simulink model "FIR_Symmetric_Ex2"  (R2025a)
settings: Solver=VariableStepAuto  StartTime=0.0  StopTime=1  RelTol=1e-3
PostLoadFcn:
  | Fs = 100000;  % Sampling Frequency
  | Fpass = 4000;              % Passband Frequency
  | Fstop = 10000;             % Stopband Frequency
  | Dpass = 0.0046051376314;   % Passband Ripple
  | Dstop = 0.00025118864315;  % Stopband Attenuation
  | dens  = 16;                % Density Factor
  | % Calculate the order from the parameters using FIRPMORD.
  | [N, Fo, Ao, W] = firpmord([Fpass, Fstop]/(Fs/2), [1 0], [Dpass, Dstop]);
  | % Calculate the coefficients using the FIRPM function.
  | coeffs = firpm(N, Fo, Ao, W, {dens});
InitFcn:
  | Fs = 100000;  % Sampling Frequency
  | Fpass = 4000;              % Passband Frequency
  | Fstop = 10000;             % Stopband Frequency
  | Dpass = 0.0046051376314;   % Passband Ripple
  | Dstop = 0.00025118864315;  % Stopband Attenuation
  | dens  = 16;                % Density Factor
  | % Calculate the order from the parameters using FIRPMORD.
  | [N, Fo, Ao, W] = firpmord([Fpass, Fstop]/(Fs/2), [1 0], [Dpass, Dstop]);
  | % Calculate the coefficients using the FIRPM function.
  | coeffs = firpm(N, Fo, Ao, W, {dens});
undefined symbols (not defined in the file): firpmord, None, S, vsva2197, xcvc1902
libraries: aieDSP x1, dspsrcs4 x1, dspmlti4 x1, vmcUtilities x1
settings Model: Creator=robg  LastModifiedBy=robg
settings DebuggingCC: UnconnectedInputMsg=warning  UnconnectedOutputMsg=warning  UnconnectedLineMsg=warning
settings ModelReferenceCC: EnableRefExpFcnMdlSchedulingChecks=on
settings RTWCC: GPUComputeCapability=3.5  DLArmComputeVersion=19.05

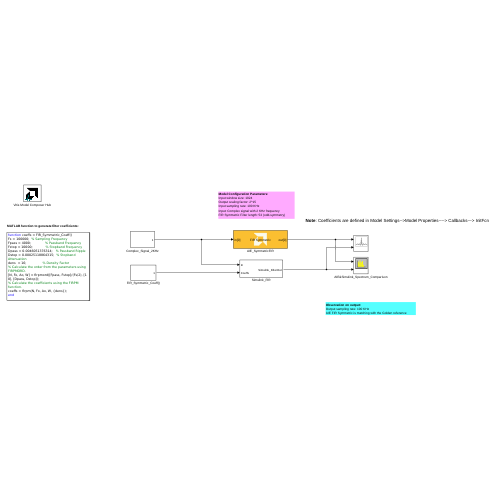
[thumbnail: Simulink's stored preview of the top-level diagram]
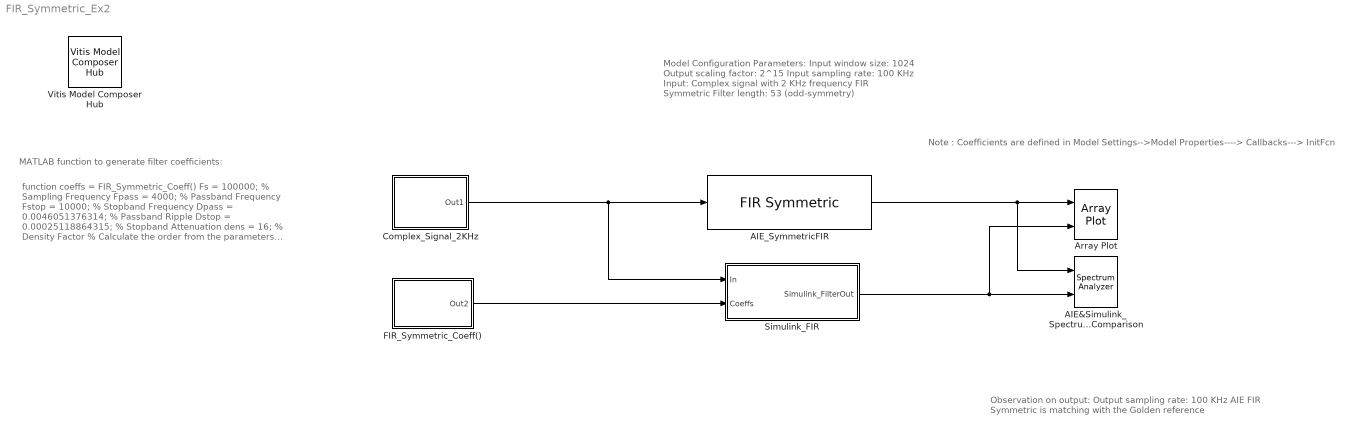
== system FIR_Symmetric_Ex2 ==
  note: Note : Coefficients are defined in Model Settings-->Model Properties----> Callbacks---> InitFcn
  note: Observation on output:
      | Output sampling rate: 100 KHz
      | AIE FIR Symmetric is matching with the Golden reference
  note: Model Configuration Parameters:
      | Input window size: 1024
      | Output scaling factor: 2^15
      | Input sampling rate: 100 KHz
      | Input: Complex signal with 2 KHz frequency
      | FIR Symmetric Filter length: 53 (odd-symmetry)
  note: MATLAB function to generate filter coefficients:
  note: function coeffs = FIR_Symmetric_Coeff()
      | Fs = 100000; % Sampling Frequency
      | Fpass = 4000; % Passband Frequency
      | Fstop = 10000; % Stopband Frequency
      | Dpass = 0.0046051376314; % Passband Ripple
      | Dstop = 0.00025118864315; % Stopband Attenuation
      | dens = 16; % Density Factor
      | % Calculate the order from the parameters using FIRPMORD.
      | [N, Fo, Ao, W] = firpmord([Fpass, Fstop]/(Fs/2), [1 0], [Dpass, Dstop]);
      | % Calculate the coefficients using the FIRPM function.
      | coeffs = firpm(N, Fo, Ao, W, {dens});
      | end
  AIE&Simulink_Spectrum_Comparison : SpectrumAnalyzer  NumInputPorts=2  WindowPosition=[439.000000,381.000000,800.000000,500.000000,]  Visible=on  ScopeFrameLocation=window  Span=99999.99999999999  StartFrequency=-49999.99999999999  StopFrequency=49999.99999999999  AveragingMethod=Exponential  YLimits=[-4.47944505,122.1232277]  ShowLegend=on  ChannelNames="[\"\"]"  AllowFFTLengthLessThanSamplesPerUpdate=on  DefaultConfigurationName=spbscopes.SpectrumAnalyzerBlockCfg
  AIE_SymmetricFIR : aieDSP/FIR Symmetric  data_type=cint16  coef_type=int16  use_coeff_reload=off  dual_ip=off  num_outputs=off  coeff=int16(coeffs(1:27)*2^15)  fir_length=53  input_window_size=1024  shift_val=15  rnd_mode=Round to positive infinity  sat_mode=0-None  casc_length=1  AIE_VARIANT=1  TP_API=0  ssr=1  blockJsonConstraints=[]  blockJsonConstraintsInternal=[]  spec=vmc_fir_sr_sym.json  SerializedMaskParamNames=[]  SerializedMaskParamValues=[]  SerializedMaskParamVisibilities=[]  block_type=FIR Symmetric  SerializedMaskParamDataypes=typename|typename|uint|uint|uint|coef_type|uint|uint|uint|uint|uint|uint|uint|uint|uint  SerializedMaskParamEnumStrArr=0|0|0|0|0|0|0|0|0|Floor,Ceiling,Round to positive infinity,Round to negative infinity,Round symmetrical to infinity,Round symmetrical to zero,Round convergent to even,Round convergent to odd|0-None,1-Asymmetric,3-Symmetric|0|0|0|0  SerializedMaskParamEnumValArr=0|0|0|0|0|0|0|0|0|0,1,2,3,4,5,6,7|0,1,3|0|0|0|0  SerializedMaskParamVectorArr=0|0|0|0|0|1|0|0|0|0|0|0|0|0|0  SerializedMaskParamKeys=TT_DATA|TT_COEFF|TP_USE_COEFF_RELOAD|TP_DUAL_IP|TP_NUM_OUTPUTS|coeff|TP_FIR_LEN|TP_INPUT_WINDOW_VSIZE|TP_SHIFT|TP_RND|TP_SAT|TP_CASC_LEN|AIE_VARIANT|TP_API|TP_SSR
  Array Plot : ArrayPlot  NumInputPorts=2  WindowPosition=[899.000000,280.000000,800.000000,500.000000,]  Visible=on  ScopeFrameLocation=window  PlotType=Line  YLimits=[-20287.625 20318.625]  ShowLegend=on
  Complex_Signal_2KHz : Subsystem
  FIR_Symmetric_Coeff() : Subsystem
  Simulink_FIR : Subsystem
  Vitis Model Composer Hub : vmcUtilities/Vitis Model Composer Hub  Tag=genX  CodeGeneration=off  StartColumn=1  NumberOfColumns=1  TargetDirectory=./code  exportDesign=off  analyzeDesign=off  validateDesignOnHw=off  ExportType=AI Engines  IpVendor=xilinx.com  IpLibrary=hls  IpVersion=1.0  IpHWLanguage=Verilog  AieCompilerOptions={}  AieSimulatorOptions={}  CreateTestbench=off  TestbenchStackSize=10  RunRtlSim=off  RunCSim=off  RunAieSim=off  enableSimulationTimeout=on  enableGraphIterations=on  AieSimTimeout=50000  AieGraphIterations=-1  RunAieSimProfiling=off  LaunchVitisAnalyzer=off  PlotOutput=off  RunX86Sim=off  X86SimTimeout=10  GenHwImage=off  GenLibadfXo=off  GenHwValidationCode=off  PlatformType=Not Specified  HwSystemType=Baremetal  HwValidationTarget=hw  ProjDevice=xcvc1902-vsva2197-1LP-e-S  ProjDevicePart=xcvc1902-vsva2197-1LP-e-S  AIEType=AIE  SamplePeriod=-1  ClockFrequency=200  DataPathParallelism=1  xilinxfamily=versalaicore  part=xcvc1902  speed=-1LP-e-S  package=vsva2197  directory=./netlist  testbench=off  incr_netlist=off  synthesis_tool=Vivado  clock_wrapper=Clock Enables  dbl_ovrd=According to Block Masks  dcm_input_clock_period=10  sysclk_period=10  simulink_period=1  eval_field=0  LogFileName=''  NThreads=4
  wires:
  FIR_Symmetric_Coeff()/1(Out2) -> Simulink_FIR/2(Coeffs)
  Simulink_FIR/1(Simulink_FilterOut) -> Array Plot/2, AIE&Simulink_Spectrum_Comparison/2
  Complex_Signal_2KHz/1(Out1) -> AIE_SymmetricFIR/1, Simulink_FIR/1(In)
  AIE_SymmetricFIR/1 -> AIE&Simulink_Spectrum_Comparison/1, Array Plot/1

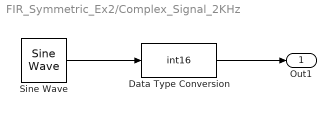
== system FIR_Symmetric_Ex2/Complex_Signal_2KHz ==
  Data Type Conversion : DataTypeConversion  OutMin=[-1]  OutMax=[1]  OutDataTypeStr=int16  ConvertRealWorld=Stored Integer (SI)  SaturateOnIntegerOverflow=off  RndMeth=Floor
  Sine Wave : dspsrcs4/Sine Wave  Amplitude=1  Frequency=2e3  Phase=0  SampleMode=Discrete  OutComplex=Complex  CompMethod=Table lookup  TableSize=Speed  SampleTime=1/100e3  SamplesPerFrame=1024  ResetState=Restart at time zero  OutputFrames=off  dataType=Fixed-point  wordLen=16  udDataType=sfix(16)  fracBitsMode=User-defined  numFracBits=14  OutDataTypeStr=fixdt(1,16,14)  LastOutDataTypeStr=fixdt(1,16,14)
  Out1 : Outport
  wires:
  Sine Wave/1 -> Data Type Conversion/1
  Data Type Conversion/1 -> Out1/1

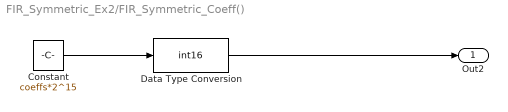
== system FIR_Symmetric_Ex2/FIR_Symmetric_Coeff() ==
  Constant : Constant  Value=coeffs*2^15
  Data Type Conversion : DataTypeConversion  OutMin=[-1]  OutMax=[1]  OutDataTypeStr=int16  ConvertRealWorld=Stored Integer (SI)  SaturateOnIntegerOverflow=off  RndMeth=Floor
  Out2 : Outport
  wires:
  Constant/1 -> Data Type Conversion/1
  Data Type Conversion/1 -> Out2/1

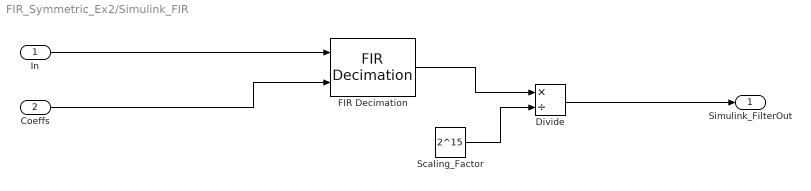
== system FIR_Symmetric_Ex2/Simulink_FIR ==
  In : Inport
  Coeffs : Inport  Port=2
  Divide : Product  Inputs=*/  OutDataTypeStr=int16
  FIR Decimation : dspmlti4/FIR Decimation  FilterSource=Input port  h=int16(firpm(63, [0;0.1;0.2;1], [1;1;0;0], [1;18.3333831245308], {16})*2^15)  D=1  filtStruct=Direct form  FilterObject=firpmord([5e3, 10e3]/(100e3/2), [1 0], [0.0046051376314, 0.0001995262315])  InputProcessing=Columns as channels (frame based)  framing=Enforce single-rate processing  AllowArbitraryInputLength=off  inputOffset=0  outputBufInitCond=0  roundingMode=Floor  overflowMode=off  firstCoeffDataTypeStr=Inherit: Same word length as input  firstCoeffMin=[]  firstCoeffMax=[]  firstCoeffLastDataTypeStr=Inherit: Same word length as input  prodOutputMode=Binary point scaling  prodOutputWordLength=32  prodOutputFracLength=0  prodOutputDataTypeStr=fixdt(1,32,0)  prodOutputLastDataTypeStr=fixdt(1,32,0)  accumMode=Binary point scaling  accumWordLength=48  accumFracLength=0  accumDataTypeStr=fixdt(1,48,0)  accumLastDataTypeStr=fixdt(1,48,0)  outputDataTypeStr=Inherit: Same as product output  outputMin=[]  outputMax=[]  outputLastDataTypeStr=Inherit: Same as product output
  Scaling_Factor : Constant  Value=2^15  OutDataTypeStr=int32
  Simulink_FilterOut : Outport
  wires:
  Scaling_Factor/1 -> Divide/2
  FIR Decimation/1 -> Divide/1
  In/1 -> FIR Decimation/1
  Divide/1 -> Simulink_FilterOut/1
  Coeffs/1 -> FIR Decimation/2
